simulink model "Act_1derivativo"  (R2017b)
settings: Solver=ode2  StartTime=0.0  StopTime=20  FixedStep=0.001  RelTol=1e-3
settings Model: Creator=Marco  LastModifiedBy=Marco

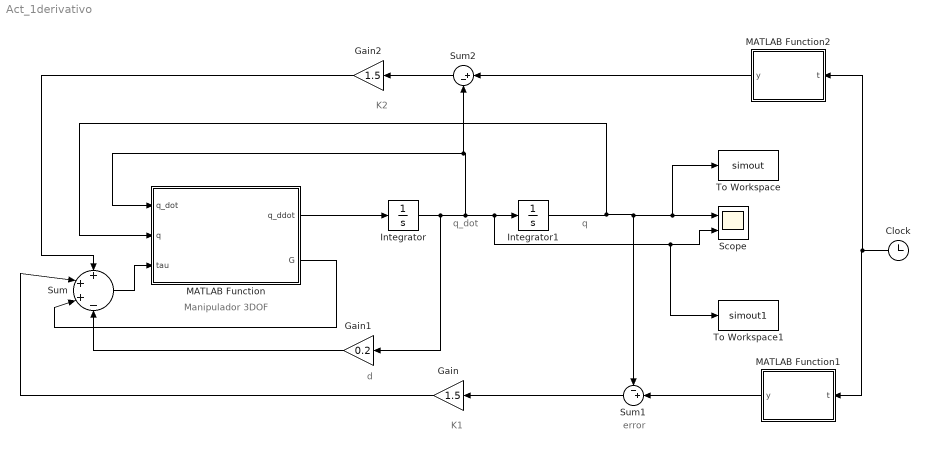
== system Act_1derivativo ==
  note: error
  note: Manipulador 3DOF
  note: d
  note: K2
  note: q
  note: q_dot
  note: K1
  Clock : Clock
  Gain : Gain  Gain=1.5
  Gain1 : Gain  Gain=0.2
  Gain2 : Gain  Gain=1.5
  Integrator : Integrator  InitialCondition=[ 0; 0]
  Integrator1 : Integrator  InitialCondition=[ pi/4; pi/2]
  MATLAB Function : MATLAB Function  TreatAsAtomicUnit=on
  MATLAB Function1 : MATLAB Function  TreatAsAtomicUnit=on
  MATLAB Function2 : MATLAB Function  TreatAsAtomicUnit=on
  Scope : Scope  NumInputPorts=2
  Sum : Sum  Inputs=+|+|+|-
  Sum1 : Sum  Inputs=-+|
  Sum2 : Sum  Inputs=|+-
  To Workspace : ToWorkspace  VariableName=simout  SaveFormat=Timeseries  SampleTime=-1
  To Workspace1 : ToWorkspace  VariableName=simout1  SaveFormat=Timeseries  SampleTime=-1
  wires:
  MATLAB Function/1(q_ddot) -> Integrator/1
  Integrator/1 -> Gain1/1, Sum2/2, MATLAB Function/1(q_dot), To Workspace1/1, Scope/2, Integrator1/1
  Integrator1/1 -> Sum1/1, To Workspace/1, Scope/1, MATLAB Function/2(q)
  Sum/1 -> MATLAB Function/3(tau)
  Sum1/1 -> Gain/1
  Gain/1 -> Sum/2
  MATLAB Function/2(G) -> Sum/3
  Gain1/1 -> Sum/4
  Sum2/1 -> Gain2/1
  Gain2/1 -> Sum/1
  Clock/1 -> MATLAB Function2/1(t), MATLAB Function1/1(t)
  MATLAB Function1/1(y) -> Sum1/2
  MATLAB Function2/1(y) -> Sum2/1

== matlab function Act_1derivativo/MATLAB Function1 ==
  data: t input; y output
function y = q(t)
y = (sin(0.5*t)+cos(2*t))*0.5;
end

== matlab function Act_1derivativo/MATLAB Function ==
  data: q_dot input; q input; q_ddot output; tau input; G output
function [q_ddot, G]= manipulador(q_dot,q,tau)
%Valores del robot
g = 9.81; %m/s^2
l_1= 0.3; %m
l_c1= 0.15; %m
l_c2= 0.15; %m
m_1= 0.2; %Kg
m_2 = 0.2; %Kg
I_1 = 0.001; %Kg*m^2
I_2 = 0.001; %Kg*m^2

%---------------------------Matriz de Inercias----------------------------%
m11 = m_1*l_c1^2+m_2*(l_c2^2+l_1^2+2*l_1*l_c2^2+2*l_1*l_c2*cos(q(2)))+I_1+I_2;
m12 = m_2*(l_c2^2+l_1*l_c2*cos(q(2)))+I_2; 
m22 = m_2*l_c2^2+I_2;

M = [m11 m12;
     m12 m22];
%----------------------------Matriz de Coriolis---------------------------%
A = -m_2*l_1*l_c2*sin(q(2));

c11 = A*q_dot(2);
c12 = A*(q_dot(1)+q_dot(2));
c21 = -A*q_dot(1);

C = [c11 c12;
     c21  0];
%----------------------------Vector de Gravedad---------------------------%
g11 = (m_1*l_c1+m_2*l_1)*g*cos(q(1))+m_2*l_c2*g*cos(q(1)+q(2));
g21 = m_2*l_c2*cos(q(1)+q(2));

G = [g11;
     g21];
 
q_ddot = M\(tau-C*q_dot-G);

== matlab function Act_1derivativo/MATLAB Function2 ==
  data: t input; y output
function y = q_dot(t)
y = (cos(t*0.5)*0.5 - 2*sin(2*t))*0.5;
end
